simulink model "threephase_matrix_converter"  (R2014a)
settings: Solver=ode23tb  StartTime=0.0  StopTime=0.1  RelTol=1e-4
PreLoadFcn:
  | Ts=2.5e-6;
InitFcn:
  | Ts=2.5e-6;
StartFcn:
  | tic;
StopFcn:
  | toc;
undefined symbols (not defined in the file or in its folder): DiscIntNeverNeededParam
libraries: powerlib x46, simulink x6
(part 1 of 2)
Description:
  | Copyright 2008 The MathWorks(TM), Inc.
settings Model: Creator=Graham Dudgeon  LastModifiedBy=cosorio
settings DataIOCC: SaveOutput=off  SaveTime=off
settings OptimizationCC: ExpressionDepthLimit=2147483647  InitFltsAndDblsToZero=on
settings DebuggingCC: SaveWithParameterizedLinksMsg=none  UnderspecifiedInitializationDetection=Classic  SignalResolutionControl=TryResolveAllWithWarning  SolverPrmCheckMsg=none  MultiTaskDSMMsg=warning  MultiTaskCondExecSysMsg=none  FcnCallInpInsideContextMsg=UseLocalSettings  StateNameClashWarn=warning
settings RTWCC: IncludeERTFirstTime=on
settings GRTTargetCC: TargetFcnLib=ansi_tfl_tmw.mat  CombineOutputUpdateFcns=off  GRTInterface=on

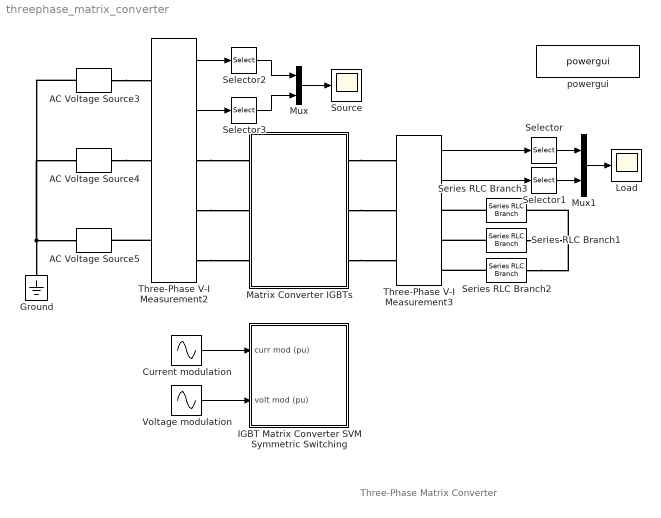
== system threephase_matrix_converter ==
  note: Three-Phase Matrix Converter
  AC Voltage Source3 : powerlib/Electrical Sources/AC Voltage Source  Amplitude=100  Phase=0  Frequency=60  SampleTime=0  Measurements=None
  AC Voltage Source4 : powerlib/Electrical Sources/AC Voltage Source  Amplitude=100  Phase=-120  Frequency=60  SampleTime=0  Measurements=None
  AC Voltage Source5 : powerlib/Electrical Sources/AC Voltage Source  Amplitude=100  Phase=120  Frequency=60  SampleTime=0  Measurements=None
  Current modulation : Sin  Amplitude=1*sqrt(2)/sqrt(3)  Frequency=2*pi*60  Phase=[0 -2*pi/3 2*pi/3]  SampleTime=0
  Ground : powerlib/Elements/Ground  LConnTagsString=a
  IGBT Matrix Converter SVM Symmetric Switching : Subsystem
  Load : Scope
      settings: YMin=-175  YMax=175  SaveName=vl1
  Matrix Converter IGBTs : Subsystem
      mask Display:
      | plot([0 10],[0 0])
      | plot([0 10],[4 4])
      | plot([0 10],[8 8])
      | plot([10 11],[8 7],[11 12.5],[7 6.5],[12 13],[6 5])
      | plot([10 11]-4,[8 7],[11 12.5]-4,[7 6.5],[12 13]-4,[6 5])
      | plot([10 11]-8,[8 7],[11 12.5]-8,[7 6.5],[12 13]-8,[6 5])
      | plot([10 11],[8 7]-4,[11 12.5],[7 6.5]-4,[12 13],[6 5]-4)
      | plot([10 11]-4,[8 7]-4,[11 12.5]-4,[7 6.5]-4,[12 13]-4,[6 5]-4)
      | plot([10 11]-8,[8 7]-4,[11 12.5]-8,[7 6.5]-4,[12 13]-8,[6 5]-4)
      | plot([10 11],[8 7]-8,[11 12.5],[7 6.5]-8,[12 13],[6 5]-8)
      | plot([10 11]-4,[8 7]-8,[11 12.5]-4,[7 6.5]-8,[12 13]-4,[6 5]-8)
      | plot([10 11]-8,[8 7]-8,[11 12.5]-8,[7 6.5]-8,[12 13]-8,[6 5]-8)
      | plot([5 5],[-5 5])
      | plot([9 9],[-5 5])
      | plot([13 13],[-5 5])
      | plot(-2,-6,15,9)
      | plot([0 0],[-5 -2])
      | plot([0.5 0.5],[-5 -2])
      | plot([0.5 1.5],[-4 -5])
      | plot([0.5 1.5],[-3 -2])
      | plot([1.5 1.5],[-5 -6])
      | plot([1.5 1.5],[-2 -1])
      | plot([1 1.5],[-4.8 -5])
      | plot([1.3 1.5],[-4.4 -5])
      | plot([-0.5 0],[-5 -5])
  Mux : Mux  Inputs=2
  Mux1 : Mux  Inputs=2
  Selector{,1..3} (4 alike) : Selector  InputPortWidth=3
  Series RLC Branch1 : powerlib/Elements/Series RLC Branch  LConnTagsString=__new0  RConnTagsString=__new0  BranchType=R  Resistance=2  Inductance=1e-3  SetiL0=off  InitialCurrent=0  Capacitance=[]  Setx0=off  InitialVoltage=0  Measurements=None
  Series RLC Branch2 : powerlib/Elements/Series RLC Branch  LConnTagsString=__new0  RConnTagsString=__new0  BranchType=R  Resistance=2  Inductance=1e-3  SetiL0=off  InitialCurrent=0  Capacitance=[]  Setx0=off  InitialVoltage=0  Measurements=None
  Series RLC Branch3 : powerlib/Elements/Series RLC Branch  LConnTagsString=__new0  RConnTagsString=__new0  BranchType=R  Resistance=2  Inductance=1e-3  SetiL0=off  InitialCurrent=0  Capacitance=[]  Setx0=off  InitialVoltage=0  Measurements=None
  Source : Scope
      settings: YMin=-100  YMax=100  SaveName=vl
  Three-Phase V-I Measurement2 : powerlib/Measurements/Three-Phase V-I Measurement  VoltageMeasurement=phase-to-ground  SetLabelV=off  LabelV=Vabc  Vpu=off  VpuLL=off  CurrentMeasurement=yes  SetLabelI=off  LabelI=Iabc  Ipu=off  Pbase=100e6  Vbase=500e3  OutputType=Complex  PhasorSimulation=off  PSBequivalent=0
  Three-Phase V-I Measurement3 : powerlib/Measurements/Three-Phase V-I Measurement  VoltageMeasurement=phase-to-phase  SetLabelV=off  LabelV=Vabc  Vpu=off  VpuLL=off  CurrentMeasurement=yes  SetLabelI=off  LabelI=Iabc  Ipu=off  Pbase=100e6  Vbase=500e3  OutputType=Complex  PhasorSimulation=off  PSBequivalent=0
  Voltage modulation : Sin  Amplitude=1*sqrt(2)/sqrt(3)  Frequency=2*pi*60  Phase=[0 -2*pi/3 2*pi/3]  SampleTime=0
  powergui : powerlib/powergui  SimulationMode=Continuous  SolverType=Tustin  SampleTime=2.5e-6  frequency=60  SPID=off  DisableSnubberDevices=on  DisableRonSwitches=off  DisableVfSwitches=off  SwTol=0  Interpol=off  DisplayEquations=off  Ts=0  methode=off  frequencyindice=60  Pbase=100e6  ErrMax=1e-4  Iterations=50  UnitsV=kV  UnitsW=MW  FunctionMessages=off  echomessages=off  HookPort=off  EnableUseOfTLC=off  x0status=blocks  RestoreLinks=warning  ResistiveCurrentMeasurement=off  Frange=[0:2:500]  Ylog=off  Xlog=on  ShowGrid=off  save=off  variable=ZData  structure=Vs  ZoomFFT=on  StartTime=1/60  cycles=1  DisplayStyle=1  fundamental=60  FreqAxis=on  MaxFrequency=10000  frequencyindicesteady=1  RmsSteady=1  display=off
  wires:
  Current modulation/1 -> IGBT Matrix Converter SVM Symmetric Switching/1(curr mod (pu))
  Voltage modulation/1 -> IGBT Matrix Converter SVM Symmetric Switching/2(volt mod (pu))
  Three-Phase V-I Measurement3/1 -> Selector/1
  Three-Phase V-I Measurement3/2 -> Selector1/1
  Selector/1 -> Mux1/1
  Three-Phase V-I Measurement2/1 -> Selector2/1
  Three-Phase V-I Measurement2/2 -> Selector3/1
  Selector2/1 -> Mux/1
  Selector3/1 -> Mux/2
  Mux/1 -> Source/1
  Selector1/1 -> Mux1/2
  Mux1/1 -> Load/1
  connections:
  AC Voltage Source4/LConn1 -- AC Voltage Source3/LConn1 -- Ground/LConn1 -- AC Voltage Source5/LConn1
  Three-Phase V-I Measurement2/RConn1 -- Matrix Converter IGBTs/LConn1
  Three-Phase V-I Measurement2/RConn3 -- Matrix Converter IGBTs/LConn3
  AC Voltage Source3/RConn1 -- Three-Phase V-I Measurement2/LConn1
  Three-Phase V-I Measurement2/LConn3 -- AC Voltage Source5/RConn1
  AC Voltage Source4/RConn1 -- Three-Phase V-I Measurement2/LConn2
  Three-Phase V-I Measurement2/RConn2 -- Matrix Converter IGBTs/LConn2
  Series RLC Branch2/RConn1 -- Series RLC Branch1/RConn1 -- Series RLC Branch3/RConn1
  Series RLC Branch3/LConn1 -- Three-Phase V-I Measurement3/RConn1
  Series RLC Branch1/LConn1 -- Three-Phase V-I Measurement3/RConn2
  Series RLC Branch2/LConn1 -- Three-Phase V-I Measurement3/RConn3
  Matrix Converter IGBTs/RConn2 -- Three-Phase V-I Measurement3/LConn2
  Matrix Converter IGBTs/RConn3 -- Three-Phase V-I Measurement3/LConn3
  Matrix Converter IGBTs/RConn1 -- Three-Phase V-I Measurement3/LConn1

== system threephase_matrix_converter/IGBT Matrix Converter SVM Symmetric Switching ==
  curr mod (pu) : Inport
  volt mod (pu) : Inport  Port=2
  SVM Inversion symmetric sequence : Subsystem  mask{switching_freq=6000}
      mask prompts: switching_freq "switching frequency (Hz)"
  SVM Rectification symmetric sequence : Subsystem  mask{switching_freq=6000}
      mask prompts: switching_freq "switching frequency (Hz)"
  Scope{1..6} (6 alike) : Scope
      Scope1 settings: TimeRange=0.1  YMin=1000  YMax=8000  SaveName=Vabc  Decimation=100
      Scope2 settings: TimeRange=0.1  YMin=1000  YMax=8000  SaveName=Vabc1  Decimation=100
      Scope3 settings: TimeRange=0.1  YMin=1000  YMax=8000  SaveName=Vabc2  Decimation=100
      Scope4 settings: TimeRange=0.1  YMin=1000  YMax=8000  SaveName=Vabc3  Decimation=100
      Scope5 settings: TimeRange=0.1  YMin=1000  YMax=8000  SaveName=Vabc4  Decimation=100
      Scope6 settings: TimeRange=0.1  YMin=1000  YMax=8000  SaveName=Vabc5  Decimation=100
  matrix converter switching : Subsystem
  matrix-converter switching count : Subsystem
  six-device switching count : Subsystem
  six-device switching count1 : Subsystem
  wires:
  SVM Inversion symmetric sequence/1(g) -> matrix converter switching/2(gI), six-device switching count1/1(pulses)
  SVM Rectification symmetric sequence/1(g) -> matrix converter switching/1(gR), six-device switching count/1(pulses)
  curr mod (pu)/1 -> SVM Rectification symmetric sequence/1(mod (pu))
  volt mod (pu)/1 -> SVM Inversion symmetric sequence/1(mod (pu))
  matrix-converter switching count/2(individual) -> Scope2/1
  matrix-converter switching count/1(total) -> Scope1/1
  matrix converter switching/1(g) -> matrix-converter switching count/1(pulses)
  six-device switching count/1(total) -> Scope3/1
  six-device switching count/2(individual) -> Scope4/1
  six-device switching count1/1(total) -> Scope5/1
  six-device switching count1/2(individual) -> Scope6/1

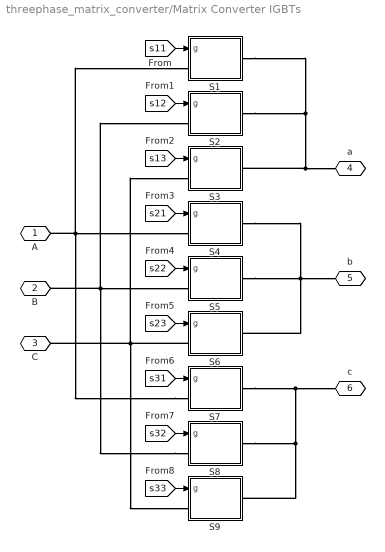
== system threephase_matrix_converter/Matrix Converter IGBTs ==
  S1 : Subsystem
  S2 : Subsystem
  S3 : Subsystem
  S4 : Subsystem
  S5 : Subsystem
  S6 : Subsystem
  S7 : Subsystem
  S8 : Subsystem
  S9 : Subsystem
  A : PMIOPort  Port=1  Side=Left
  B : PMIOPort  Port=2  Side=Left
  C : PMIOPort  Port=3  Side=Left
  a : PMIOPort  Port=4  Side=Right
  b : PMIOPort  Port=5  Side=Right
  c : PMIOPort  Port=6  Side=Right
  wires:
  [s33] -> S9/1(g)
  [s32] -> S8/1(g)
  [s31] -> S7/1(g)
  [s23] -> S6/1(g)
  [s22] -> S5/1(g)
  [s21] -> S4/1(g)
  [s13] -> S3/1(g)
  [s12] -> S2/1(g)
  [s11] -> S1/1(g)
  connections:
  c/RConn1 -- S7/RConn1 -- S9/RConn1 -- S8/RConn1
  S6/RConn1 -- S4/RConn1 -- b/RConn1 -- S5/RConn1
  C/RConn1 -- S3/LConn1 -- S6/LConn1 -- S9/LConn1
  S8/LConn1 -- S2/LConn1 -- B/RConn1 -- S5/LConn1
  S3/RConn1 -- S1/RConn1 -- S2/RConn1 -- a/RConn1
  S7/LConn1 -- A/RConn1 -- S1/LConn1 -- S4/LConn1

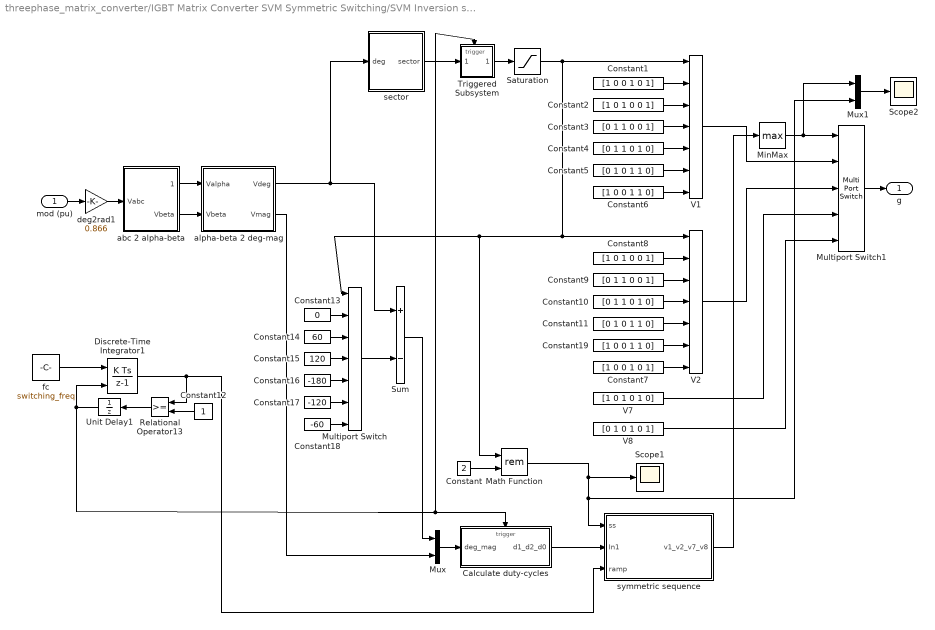
== system threephase_matrix_converter/IGBT Matrix Converter SVM Symmetric Switching/SVM Inversion symmetric sequence ==
  mod (pu) : Inport
  Calculate duty-cycles : Subsystem  TreatAsAtomicUnit=on
  Constant : Constant  Value=2
  Constant1 : Constant  Value=[1 0 0 1 0 1]
  Constant10 : Constant  Value=[0 1 1 0 1 0]
  Constant11 : Constant  Value=[0 1 0 1 1 0]
  Constant12 : Constant
  Constant13 : Constant  Value=0
  Constant14 : Constant  Value=60
  Constant15 : Constant  Value=120
  Constant16 : Constant  Value=-180
  Constant17 : Constant  Value=-120
  Constant18 : Constant  Value=-60
  Constant19 : Constant  Value=[1 0 0 1 1 0]
  Constant2 : Constant  Value=[1 0 1 0 0 1]
  Constant3 : Constant  Value=[0 1 1 0 0 1]
  Constant4 : Constant  Value=[0 1 1 0 1 0]
  Constant5 : Constant  Value=[0 1 0 1 1 0]
  Constant6 : Constant  Value=[1 0 0 1 1 0]
  Constant7 : Constant  Value=[1 0 0 1 0 1]
  Constant8 : Constant  Value=[1 0 1 0 0 1]
  Constant9 : Constant  Value=[0 1 1 0 0 1]
  Discrete-Time Integrator1 : DiscreteIntegrator  ExternalReset=rising  SampleTime=Ts  ICPrevOutput=DiscIntNeverNeededParam  ICPrevScaledInput=DiscIntNeverNeededParam
  Math Function : Math  Operator=rem  SaturateOnIntegerOverflow=on
  MinMax : MinMax  Function=max
  Multiport Switch : MultiPortSwitch  Inputs=6
  Multiport Switch1 : MultiPortSwitch  Inputs=4
  Mux : Mux  Inputs=2
  Mux1 : Mux  Inputs=2
  Relational Operator13 : RelationalOperator  InputSameDT=on
  Saturation : Saturate  UpperLimit=6  LowerLimit=1
  Scope1 : Scope
      settings: YMin=-0.1  YMax=4.1  SaveName=Iabc1
  Scope2 : Scope
      settings: YMin=-0.1  YMax=4.1  SaveName=Iabc2
  Sum : Sum  Inputs=+-
  Triggered Subsystem : Subsystem  TreatAsAtomicUnit=on
  Unit Delay1 : UnitDelay  SampleTime=Ts
  V1 : MultiPortSwitch  Inputs=6
  V2 : MultiPortSwitch  Inputs=6
  V7 : Constant  Value=[1 0 1 0 1 0]
  V8 : Constant  Value=[0 1 0 1 0 1]
  abc 2 alpha-beta : Subsystem
  alpha-beta 2 deg-mag : Subsystem
  deg2rad1 : Gain  Gain=0.866
  fc : Constant  Value=switching_freq
  sector : Subsystem
  symmetric sequence : Subsystem
  g : Outport
  wires:
  Mux1/1 -> Scope2/1
  Math Function/1 -> Mux1/2, symmetric sequence/1(ss), Scope1/1
  symmetric sequence/1(v1_v2_v7_v8) -> MinMax/1
  Constant/1 -> Math Function/2
  deg2rad1/1 -> abc 2 alpha-beta/1(Vabc)
  Triggered Subsystem/1(Out1) -> Saturation/1
  sector/1(sector) -> Triggered Subsystem/1(In1)
  Saturation/1 -> V1/1, Math Function/1, Multiport Switch/1, V2/1
  Unit Delay1/1 -> Calculate duty-cycles/Trigger, Triggered Subsystem/Trigger, Discrete-Time Integrator1/2
  Multiport Switch1/1 -> g/1
  MinMax/1 -> Mux1/1, Multiport Switch1/1
  V8/1 -> Multiport Switch1/5
  V7/1 -> Multiport Switch1/4
  V2/1 -> Multiport Switch1/3
  V1/1 -> Multiport Switch1/2
  Constant7/1 -> V2/7
  Constant6/1 -> V1/7
  Constant2/1 -> V1/3
  Constant19/1 -> V2/6
  Constant11/1 -> V2/5
  Constant10/1 -> V2/4
  Constant9/1 -> V2/3
  Constant8/1 -> V2/2
  Constant5/1 -> V1/6
  Constant4/1 -> V1/5
  Constant3/1 -> V1/4
  Constant1/1 -> V1/2
  Sum/1 -> Mux/1
  Multiport Switch/1 -> Sum/2
  Constant18/1 -> Multiport Switch/7
  Constant17/1 -> Multiport Switch/6
  Constant16/1 -> Multiport Switch/5
  Constant15/1 -> Multiport Switch/4
  Constant14/1 -> Multiport Switch/3
  Constant13/1 -> Multiport Switch/2
  Calculate duty-cycles/1(d1_d2_d0) -> symmetric sequence/2(In1)
  abc 2 alpha-beta/2(Vbeta) -> alpha-beta 2 deg-mag/2(Vbeta)
  abc 2 alpha-beta/1(Valpha) -> alpha-beta 2 deg-mag/1(Valpha)
  Mux/1 -> Calculate duty-cycles/1(deg_mag)
  fc/1 -> Discrete-Time Integrator1/1
  Discrete-Time Integrator1/1 -> symmetric sequence/3(ramp), Relational Operator13/1
  Constant12/1 -> Relational Operator13/2
  Relational Operator13/1 -> Unit Delay1/1
  alpha-beta 2 deg-mag/2(Vmag) -> Mux/2
  alpha-beta 2 deg-mag/1(Vdeg) -> sector/1(deg), Sum/1
  mod (pu)/1 -> deg2rad1/1

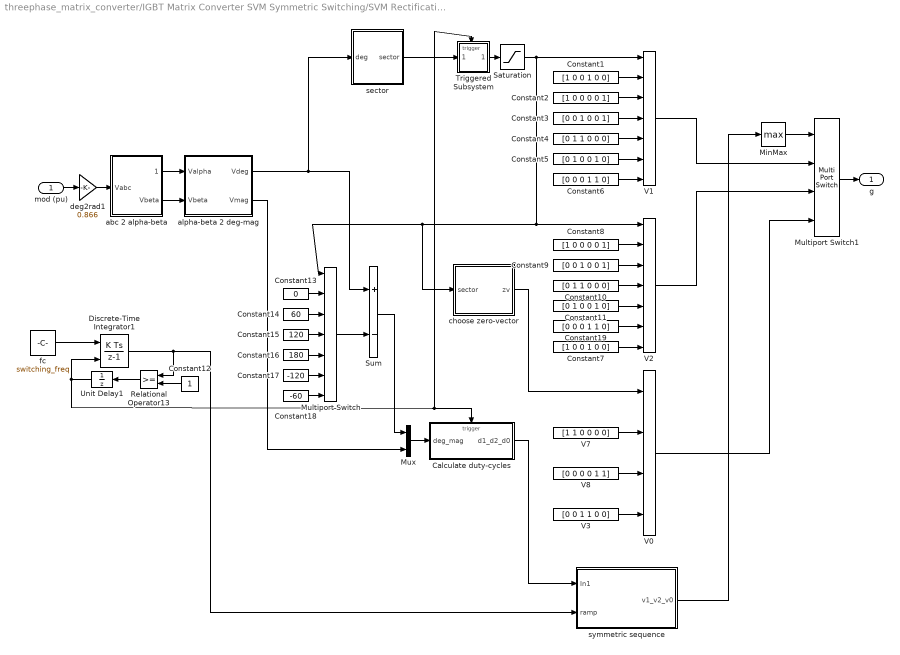
== system threephase_matrix_converter/IGBT Matrix Converter SVM Symmetric Switching/SVM Rectification symmetric sequence ==
  mod (pu) : Inport
  Calculate duty-cycles : Subsystem  TreatAsAtomicUnit=on
  Constant1 : Constant  Value=[1 0 0 1 0 0]
  Constant10 : Constant  Value=[0 1 1 0 0 0]
  Constant11 : Constant  Value=[0 1 0 0 1 0]
  Constant12 : Constant
  Constant13 : Constant  Value=0
  Constant14 : Constant  Value=60
  Constant15 : Constant  Value=120
  Constant16 : Constant  Value=180
  Constant17 : Constant  Value=-120
  Constant18 : Constant  Value=-60
  Constant19 : Constant  Value=[0 0 0 1 1 0]
  Constant2 : Constant  Value=[1 0 0 0 0 1]
  Constant3 : Constant  Value=[0 0 1 0 0 1]
  Constant4 : Constant  Value=[0 1 1 0 0 0]
  Constant5 : Constant  Value=[0 1 0 0 1 0]
  Constant6 : Constant  Value=[0 0 0 1 1 0]
  Constant7 : Constant  Value=[1 0 0 1 0 0]
  Constant8 : Constant  Value=[1 0 0 0 0 1]
  Constant9 : Constant  Value=[0 0 1 0 0 1]
  Discrete-Time Integrator1 : DiscreteIntegrator  ExternalReset=rising  SampleTime=Ts  ICPrevOutput=DiscIntNeverNeededParam  ICPrevScaledInput=DiscIntNeverNeededParam
  MinMax : MinMax  Function=max
  Multiport Switch : MultiPortSwitch  Inputs=6
  Multiport Switch1 : MultiPortSwitch
  Mux : Mux  Inputs=2
  Relational Operator13 : RelationalOperator  InputSameDT=on
  Saturation : Saturate  UpperLimit=6  LowerLimit=1
  Sum : Sum  Inputs=+-
  Triggered Subsystem : Subsystem  TreatAsAtomicUnit=on
  Unit Delay1 : UnitDelay  SampleTime=Ts
  V0 : MultiPortSwitch
  V1 : MultiPortSwitch  Inputs=6
  V2 : MultiPortSwitch  Inputs=6
  V3 : Constant  Value=[0 0 1 1 0 0]
  V7 : Constant  Value=[1 1 0 0 0 0]
  V8 : Constant  Value=[0 0 0 0 1 1]
  abc 2 alpha-beta : Subsystem
  alpha-beta 2 deg-mag : Subsystem
  choose zero-vector : Subsystem
  deg2rad1 : Gain  Gain=0.866
  fc : Constant  Value=switching_freq
  sector : Subsystem
  symmetric sequence : Subsystem
  g : Outport
  wires:
  deg2rad1/1 -> abc 2 alpha-beta/1(Vabc)
  Saturation/1 -> V1/1, V2/1, Multiport Switch/1, choose zero-vector/1(sector)
  Triggered Subsystem/1(Out1) -> Saturation/1
  sector/1(sector) -> Triggered Subsystem/1(In1)
  MinMax/1 -> Multiport Switch1/1
  Unit Delay1/1 -> Discrete-Time Integrator1/2, Calculate duty-cycles/Trigger, Triggered Subsystem/Trigger
  Multiport Switch1/1 -> g/1
  symmetric sequence/1(v1_v2_v0) -> MinMax/1
  V2/1 -> Multiport Switch1/3
  V1/1 -> Multiport Switch1/2
  Constant7/1 -> V2/7
  Constant6/1 -> V1/7
  Constant2/1 -> V1/3
  Constant19/1 -> V2/6
  Constant11/1 -> V2/5
  Constant10/1 -> V2/4
  Constant9/1 -> V2/3
  Constant8/1 -> V2/2
  Constant5/1 -> V1/6
  Constant4/1 -> V1/5
  Constant3/1 -> V1/4
  Constant1/1 -> V1/2
  Sum/1 -> Mux/1
  Multiport Switch/1 -> Sum/2
  Constant18/1 -> Multiport Switch/7
  Constant17/1 -> Multiport Switch/6
  Constant16/1 -> Multiport Switch/5
  Constant15/1 -> Multiport Switch/4
  Constant14/1 -> Multiport Switch/3
  Constant13/1 -> Multiport Switch/2
  Calculate duty-cycles/1(d1_d2_d0) -> symmetric sequence/1(In1)
  abc 2 alpha-beta/2(Vbeta) -> alpha-beta 2 deg-mag/2(Vbeta)
  abc 2 alpha-beta/1(Valpha) -> alpha-beta 2 deg-mag/1(Valpha)
  Mux/1 -> Calculate duty-cycles/1(deg_mag)
  fc/1 -> Discrete-Time Integrator1/1
  Discrete-Time Integrator1/1 -> Relational Operator13/1, symmetric sequence/2(ramp)
  Constant12/1 -> Relational Operator13/2
  Relational Operator13/1 -> Unit Delay1/1
  alpha-beta 2 deg-mag/2(Vmag) -> Mux/2
  alpha-beta 2 deg-mag/1(Vdeg) -> sector/1(deg), Sum/1
  mod (pu)/1 -> deg2rad1/1
  V7/1 -> V0/2
  V8/1 -> V0/3
  V3/1 -> V0/4
  V0/1 -> Multiport Switch1/4
  choose zero-vector/1(zv) -> V0/1

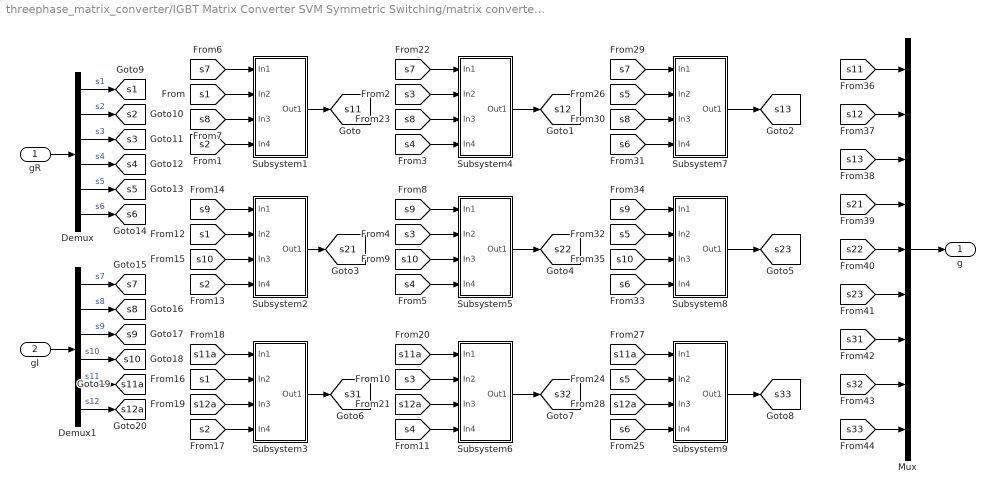
== system threephase_matrix_converter/IGBT Matrix Converter SVM Symmetric Switching/matrix converter switching ==
  gR : Inport
  gI : Inport  Port=2
  Demux : Demux  Outputs=6
  Demux1 : Demux  Outputs=6
  Mux : Mux  Inputs=9
  Subsystem1 : Subsystem
  Subsystem2 : Subsystem
  Subsystem3 : Subsystem
  Subsystem4 : Subsystem
  Subsystem5 : Subsystem
  Subsystem6 : Subsystem
  Subsystem7 : Subsystem
  Subsystem8 : Subsystem
  Subsystem9 : Subsystem
  g : Outport
  tag scope: s10=global, s11=global, s11a=global, s12=global, s12a=global, s13=global, s1=global, s21=global, s22=global, s23=global, s2=global, s31=global, s32=global, s33=global, s3=global, s4=global, s5=global, s6=global, s7=global, s8=global, s9=global
  wires:
  Demux/4 -> [s4]  "s4"
  Demux1/6 -> [s12a]  "s12"
  gR/1 -> Demux/1
  gI/1 -> Demux1/1
  Demux/1 -> [s1]  "s1"
  Demux1/5 -> [s11a]  "s11"
  Demux1/4 -> [s10]  "s10"
  Demux1/3 -> [s9]  "s9"
  Demux1/2 -> [s8]  "s8"
  Demux1/1 -> [s7]  "s7"
  Demux/2 -> [s2]  "s2"
  Demux/3 -> [s3]  "s3"
  Demux/5 -> [s5]  "s5"
  Demux/6 -> [s6]  "s6"
  [s7] -> Subsystem1/1(In1)
  [s1] -> Subsystem1/2(In2)
  [s8] -> Subsystem1/3(In3)
  [s2] -> Subsystem1/4(In4)
  [s9] -> Subsystem2/1(In1)
  [s1] -> Subsystem2/2(In2)
  [s10] -> Subsystem2/3(In3)
  [s2] -> Subsystem2/4(In4)
  [s11a] -> Subsystem3/1(In1)
  [s1] -> Subsystem3/2(In2)
  [s12a] -> Subsystem3/3(In3)
  [s2] -> Subsystem3/4(In4)
  [s7] -> Subsystem4/1(In1)
  [s3] -> Subsystem4/2(In2)
  [s8] -> Subsystem4/3(In3)
  [s4] -> Subsystem4/4(In4)
  [s9] -> Subsystem5/1(In1)
  [s3] -> Subsystem5/2(In2)
  [s10] -> Subsystem5/3(In3)
  [s4] -> Subsystem5/4(In4)
  [s11a] -> Subsystem6/1(In1)
  [s3] -> Subsystem6/2(In2)
  [s12a] -> Subsystem6/3(In3)
  [s4] -> Subsystem6/4(In4)
  [s7] -> Subsystem7/1(In1)
  [s5] -> Subsystem7/2(In2)
  [s8] -> Subsystem7/3(In3)
  [s6] -> Subsystem7/4(In4)
  [s9] -> Subsystem8/1(In1)
  [s5] -> Subsystem8/2(In2)
  [s10] -> Subsystem8/3(In3)
  [s6] -> Subsystem8/4(In4)
  [s11a] -> Subsystem9/1(In1)
  [s5] -> Subsystem9/2(In2)
  [s12a] -> Subsystem9/3(In3)
  [s6] -> Subsystem9/4(In4)
  Subsystem1/1(Out1) -> [s11]
  Subsystem4/1(Out1) -> [s12]
  Subsystem7/1(Out1) -> [s13]
  Subsystem2/1(Out1) -> [s21]
  Subsystem5/1(Out1) -> [s22]
  Subsystem8/1(Out1) -> [s23]
  Subsystem3/1(Out1) -> [s31]
  Subsystem6/1(Out1) -> [s32]
  Subsystem9/1(Out1) -> [s33]
  [s11] -> Mux/1
  [s12] -> Mux/2
  [s13] -> Mux/3
  [s21] -> Mux/4
  [s22] -> Mux/5
  [s23] -> Mux/6
  [s31] -> Mux/7
  [s32] -> Mux/8
  [s33] -> Mux/9
  Mux/1 -> g/1

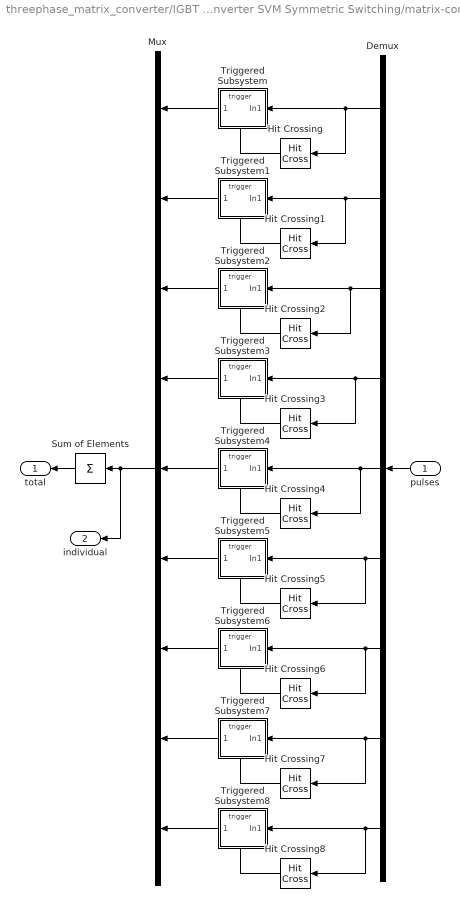
== system threephase_matrix_converter/IGBT Matrix Converter SVM Symmetric Switching/matrix-converter switching count ==
  pulses : Inport
  Demux : Demux  Outputs=9
  Hit Crossing{,1..8} (9 alike) : HitCross  HitCrossingDirection=rising
  Mux : Mux  Inputs=9
  Sum of Elements : Sum  Inputs=+
  Triggered Subsystem : Subsystem  TreatAsAtomicUnit=on
  Triggered Subsystem1 : Subsystem  TreatAsAtomicUnit=on
  Triggered Subsystem2 : Subsystem  TreatAsAtomicUnit=on
  Triggered Subsystem3 : Subsystem  TreatAsAtomicUnit=on
  Triggered Subsystem4 : Subsystem  TreatAsAtomicUnit=on
  Triggered Subsystem5 : Subsystem  TreatAsAtomicUnit=on
  Triggered Subsystem6 : Subsystem  TreatAsAtomicUnit=on
  Triggered Subsystem7 : Subsystem  TreatAsAtomicUnit=on
  Triggered Subsystem8 : Subsystem  TreatAsAtomicUnit=on
  total : Outport
  individual : Outport  Port=2
  wires:
  pulses/1 -> Demux/1
  Sum of Elements/1 -> total/1
  Mux/1 -> individual/1, Sum of Elements/1
  Demux/6 -> Triggered Subsystem5/1(In1), Hit Crossing5/1
  Hit Crossing5/1 -> Triggered Subsystem5/Trigger
  Triggered Subsystem5/1(Out1) -> Mux/6
  Demux/5 -> Triggered Subsystem4/1(In1), Hit Crossing4/1
  Hit Crossing4/1 -> Triggered Subsystem4/Trigger
  Triggered Subsystem4/1(Out1) -> Mux/5
  Demux/4 -> Triggered Subsystem3/1(In1), Hit Crossing3/1
  Hit Crossing3/1 -> Triggered Subsystem3/Trigger
  Triggered Subsystem3/1(Out1) -> Mux/4
  Demux/3 -> Triggered Subsystem2/1(In1), Hit Crossing2/1
  Hit Crossing2/1 -> Triggered Subsystem2/Trigger
  Triggered Subsystem2/1(Out1) -> Mux/3
  Demux/2 -> Triggered Subsystem1/1(In1), Hit Crossing1/1
  Hit Crossing1/1 -> Triggered Subsystem1/Trigger
  Triggered Subsystem1/1(Out1) -> Mux/2
  Demux/1 -> Triggered Subsystem/1(In1), Hit Crossing/1
  Hit Crossing/1 -> Triggered Subsystem/Trigger
  Triggered Subsystem/1(Out1) -> Mux/1
  Demux/7 -> Triggered Subsystem6/1(In1), Hit Crossing6/1
  Hit Crossing6/1 -> Triggered Subsystem6/Trigger
  Triggered Subsystem6/1(Out1) -> Mux/7
  Demux/8 -> Triggered Subsystem7/1(In1), Hit Crossing7/1
  Hit Crossing7/1 -> Triggered Subsystem7/Trigger
  Triggered Subsystem7/1(Out1) -> Mux/8
  Demux/9 -> Triggered Subsystem8/1(In1), Hit Crossing8/1
  Hit Crossing8/1 -> Triggered Subsystem8/Trigger
  Triggered Subsystem8/1(Out1) -> Mux/9

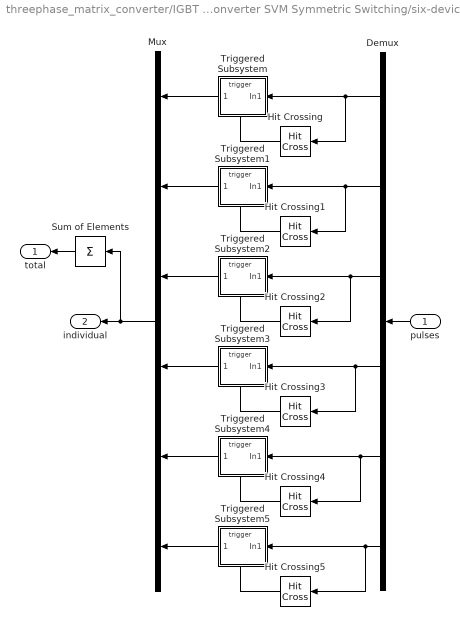
== system threephase_matrix_converter/IGBT Matrix Converter SVM Symmetric Switching/six-device switching count ==
  pulses : Inport
  Demux : Demux  Outputs=6
  Hit Crossing{,1..5} (6 alike) : HitCross  HitCrossingDirection=rising
  Mux : Mux  Inputs=6
  Sum of Elements : Sum  Inputs=+
  Triggered Subsystem : Subsystem  TreatAsAtomicUnit=on
  Triggered Subsystem1 : Subsystem  TreatAsAtomicUnit=on
  Triggered Subsystem2 : Subsystem  TreatAsAtomicUnit=on
  Triggered Subsystem3 : Subsystem  TreatAsAtomicUnit=on
  Triggered Subsystem4 : Subsystem  TreatAsAtomicUnit=on
  Triggered Subsystem5 : Subsystem  TreatAsAtomicUnit=on
  total : Outport
  individual : Outport  Port=2
  wires:
  pulses/1 -> Demux/1
  Sum of Elements/1 -> total/1
  Mux/1 -> individual/1, Sum of Elements/1
  Demux/6 -> Triggered Subsystem5/1(In1), Hit Crossing5/1
  Hit Crossing5/1 -> Triggered Subsystem5/Trigger
  Triggered Subsystem5/1(Out1) -> Mux/6
  Demux/5 -> Triggered Subsystem4/1(In1), Hit Crossing4/1
  Hit Crossing4/1 -> Triggered Subsystem4/Trigger
  Triggered Subsystem4/1(Out1) -> Mux/5
  Demux/4 -> Triggered Subsystem3/1(In1), Hit Crossing3/1
  Hit Crossing3/1 -> Triggered Subsystem3/Trigger
  Triggered Subsystem3/1(Out1) -> Mux/4
  Demux/3 -> Triggered Subsystem2/1(In1), Hit Crossing2/1
  Hit Crossing2/1 -> Triggered Subsystem2/Trigger
  Triggered Subsystem2/1(Out1) -> Mux/3
  Demux/2 -> Triggered Subsystem1/1(In1), Hit Crossing1/1
  Hit Crossing1/1 -> Triggered Subsystem1/Trigger
  Triggered Subsystem1/1(Out1) -> Mux/2
  Demux/1 -> Triggered Subsystem/1(In1), Hit Crossing/1
  Hit Crossing/1 -> Triggered Subsystem/Trigger
  Triggered Subsystem/1(Out1) -> Mux/1

== system threephase_matrix_converter/IGBT Matrix Converter SVM Symmetric Switching/six-device switching count1 ==
  pulses : Inport
  Demux : Demux  Outputs=6
  Hit Crossing{,1..5} (6 alike) : HitCross  HitCrossingDirection=rising
  Mux : Mux  Inputs=6
  Sum of Elements : Sum  Inputs=+
  Triggered Subsystem : Subsystem  TreatAsAtomicUnit=on
  Triggered Subsystem1 : Subsystem  TreatAsAtomicUnit=on
  Triggered Subsystem2 : Subsystem  TreatAsAtomicUnit=on
  Triggered Subsystem3 : Subsystem  TreatAsAtomicUnit=on
  Triggered Subsystem4 : Subsystem  TreatAsAtomicUnit=on
  Triggered Subsystem5 : Subsystem  TreatAsAtomicUnit=on
  total : Outport
  individual : Outport  Port=2
  wires:
  Triggered Subsystem/1(Out1) -> Mux/1
  Hit Crossing/1 -> Triggered Subsystem/Trigger
  Demux/1 -> Hit Crossing/1, Triggered Subsystem/1(In1)
  Triggered Subsystem1/1(Out1) -> Mux/2
  Hit Crossing1/1 -> Triggered Subsystem1/Trigger
  Demux/2 -> Hit Crossing1/1, Triggered Subsystem1/1(In1)
  Triggered Subsystem2/1(Out1) -> Mux/3
  Hit Crossing2/1 -> Triggered Subsystem2/Trigger
  Demux/3 -> Hit Crossing2/1, Triggered Subsystem2/1(In1)
  Triggered Subsystem3/1(Out1) -> Mux/4
  Hit Crossing3/1 -> Triggered Subsystem3/Trigger
  Demux/4 -> Hit Crossing3/1, Triggered Subsystem3/1(In1)
  Triggered Subsystem4/1(Out1) -> Mux/5
  Hit Crossing4/1 -> Triggered Subsystem4/Trigger
  Demux/5 -> Hit Crossing4/1, Triggered Subsystem4/1(In1)
  Triggered Subsystem5/1(Out1) -> Mux/6
  Hit Crossing5/1 -> Triggered Subsystem5/Trigger
  Demux/6 -> Hit Crossing5/1, Triggered Subsystem5/1(In1)
  Mux/1 -> Sum of Elements/1, individual/1
  Sum of Elements/1 -> total/1
  pulses/1 -> Demux/1

== system threephase_matrix_converter/Matrix Converter IGBTs/S1 ==
  g : Inport
  Diode : powerlib/Power Electronics/Diode  Ron=0.001  Lon=0  Vf=0  IC=0  UseSnubber=off  Rs=1e4  Cs=250e-9  Measurements=off
  Diode1 : powerlib/Power Electronics/Diode  Ron=0.001  Lon=0  Vf=0  IC=0  UseSnubber=off  Rs=1e4  Cs=250e-9  Measurements=off
  IGBT1 : powerlib/Power Electronics/IGBT  Ron=0.001  Lon=0  Vf=1  Tf=1e-6  Tt=2e-6  IC=0  Rs=1e5  Cs=inf  Measurements=off
  IGBT2 : powerlib/Power Electronics/IGBT  Ron=0.001  Lon=0  Vf=1  Tf=1e-6  Tt=2e-6  IC=0  Rs=1e5  Cs=inf  Measurements=off
  + : PMIOPort  Port=1  Side=Left
  - : PMIOPort  Port=2  Side=Right
  wires:
  g/1 -> IGBT2/1, IGBT1/1
  connections:
  IGBT2/LConn1 -- Diode/RConn1 -- +/RConn1
  IGBT1/LConn1 -- Diode1/RConn1 -- -/RConn1
  IGBT2/RConn1 -- IGBT1/RConn1 -- Diode/LConn1 -- Diode1/LConn1

== system threephase_matrix_converter/Matrix Converter IGBTs/S2 ==
  g : Inport
  Diode : powerlib/Power Electronics/Diode  Ron=0.001  Lon=0  Vf=0  IC=0  UseSnubber=off  Rs=1e4  Cs=250e-9  Measurements=off
  Diode1 : powerlib/Power Electronics/Diode  Ron=0.001  Lon=0  Vf=0  IC=0  UseSnubber=off  Rs=1e4  Cs=250e-9  Measurements=off
  IGBT1 : powerlib/Power Electronics/IGBT  Ron=0.001  Lon=0  Vf=1  Tf=1e-6  Tt=2e-6  IC=0  Rs=1e5  Cs=inf  Measurements=off
  IGBT2 : powerlib/Power Electronics/IGBT  Ron=0.001  Lon=0  Vf=1  Tf=1e-6  Tt=2e-6  IC=0  Rs=1e5  Cs=inf  Measurements=off
  + : PMIOPort  Port=1  Side=Left
  - : PMIOPort  Port=2  Side=Right
  wires:
  g/1 -> IGBT1/1, IGBT2/1
  connections:
  Diode1/LConn1 -- IGBT1/RConn1 -- IGBT2/RConn1 -- Diode/LConn1
  Diode1/RConn1 -- IGBT1/LConn1 -- -/RConn1
  Diode/RConn1 -- IGBT2/LConn1 -- +/RConn1

== system threephase_matrix_converter/Matrix Converter IGBTs/S3 ==
  g : Inport
  Diode : powerlib/Power Electronics/Diode  Ron=0.001  Lon=0  Vf=0  IC=0  UseSnubber=off  Rs=1e4  Cs=250e-9  Measurements=off
  Diode1 : powerlib/Power Electronics/Diode  Ron=0.001  Lon=0  Vf=0  IC=0  UseSnubber=off  Rs=1e4  Cs=250e-9  Measurements=off
  IGBT1 : powerlib/Power Electronics/IGBT  Ron=0.001  Lon=0  Vf=1  Tf=1e-6  Tt=2e-6  IC=0  Rs=1e5  Cs=inf  Measurements=off
  IGBT2 : powerlib/Power Electronics/IGBT  Ron=0.001  Lon=0  Vf=1  Tf=1e-6  Tt=2e-6  IC=0  Rs=1e5  Cs=inf  Measurements=off
  + : PMIOPort  Port=1  Side=Left
  - : PMIOPort  Port=2  Side=Right
  wires:
  g/1 -> IGBT2/1, IGBT1/1
  connections:
  +/RConn1 -- IGBT2/LConn1 -- Diode/RConn1
  -/RConn1 -- IGBT1/LConn1 -- Diode1/RConn1
  Diode/LConn1 -- IGBT2/RConn1 -- IGBT1/RConn1 -- Diode1/LConn1

== system threephase_matrix_converter/Matrix Converter IGBTs/S4 ==
  g : Inport
  Diode : powerlib/Power Electronics/Diode  Ron=0.001  Lon=0  Vf=0  IC=0  UseSnubber=off  Rs=1e4  Cs=250e-9  Measurements=off
  Diode1 : powerlib/Power Electronics/Diode  Ron=0.001  Lon=0  Vf=0  IC=0  UseSnubber=off  Rs=1e4  Cs=250e-9  Measurements=off
  IGBT1 : powerlib/Power Electronics/IGBT  Ron=0.001  Lon=0  Vf=1  Tf=1e-6  Tt=2e-6  IC=0  Rs=1e5  Cs=inf  Measurements=off
  IGBT2 : powerlib/Power Electronics/IGBT  Ron=0.001  Lon=0  Vf=1  Tf=1e-6  Tt=2e-6  IC=0  Rs=1e5  Cs=inf  Measurements=off
  + : PMIOPort  Port=1  Side=Left
  - : PMIOPort  Port=2  Side=Right
  wires:
  g/1 -> IGBT1/1, IGBT2/1
  connections:
  Diode1/LConn1 -- IGBT1/RConn1 -- IGBT2/RConn1 -- Diode/LConn1
  Diode1/RConn1 -- IGBT1/LConn1 -- -/RConn1
  Diode/RConn1 -- IGBT2/LConn1 -- +/RConn1

== system threephase_matrix_converter/Matrix Converter IGBTs/S5 ==
  g : Inport
  Diode : powerlib/Power Electronics/Diode  Ron=0.001  Lon=0  Vf=0  IC=0  UseSnubber=off  Rs=1e4  Cs=250e-9  Measurements=off
  Diode1 : powerlib/Power Electronics/Diode  Ron=0.001  Lon=0  Vf=0  IC=0  UseSnubber=off  Rs=1e4  Cs=250e-9  Measurements=off
  IGBT1 : powerlib/Power Electronics/IGBT  Ron=0.001  Lon=0  Vf=1  Tf=1e-6  Tt=2e-6  IC=0  Rs=1e5  Cs=inf  Measurements=off
  IGBT2 : powerlib/Power Electronics/IGBT  Ron=0.001  Lon=0  Vf=1  Tf=1e-6  Tt=2e-6  IC=0  Rs=1e5  Cs=inf  Measurements=off
  + : PMIOPort  Port=1  Side=Left
  - : PMIOPort  Port=2  Side=Right
  wires:
  g/1 -> IGBT2/1, IGBT1/1
  connections:
  +/RConn1 -- IGBT2/LConn1 -- Diode/RConn1
  -/RConn1 -- IGBT1/LConn1 -- Diode1/RConn1
  Diode/LConn1 -- IGBT2/RConn1 -- IGBT1/RConn1 -- Diode1/LConn1

== system threephase_matrix_converter/Matrix Converter IGBTs/S6 ==
  g : Inport
  Diode : powerlib/Power Electronics/Diode  Ron=0.001  Lon=0  Vf=0  IC=0  UseSnubber=off  Rs=1e4  Cs=250e-9  Measurements=off
  Diode1 : powerlib/Power Electronics/Diode  Ron=0.001  Lon=0  Vf=0  IC=0  UseSnubber=off  Rs=1e4  Cs=250e-9  Measurements=off
  IGBT1 : powerlib/Power Electronics/IGBT  Ron=0.001  Lon=0  Vf=1  Tf=1e-6  Tt=2e-6  IC=0  Rs=1e5  Cs=inf  Measurements=off
  IGBT2 : powerlib/Power Electronics/IGBT  Ron=0.001  Lon=0  Vf=1  Tf=1e-6  Tt=2e-6  IC=0  Rs=1e5  Cs=inf  Measurements=off
  + : PMIOPort  Port=1  Side=Left
  - : PMIOPort  Port=2  Side=Right
  wires:
  g/1 -> IGBT1/1, IGBT2/1
  connections:
  Diode1/LConn1 -- IGBT1/RConn1 -- IGBT2/RConn1 -- Diode/LConn1
  Diode1/RConn1 -- IGBT1/LConn1 -- -/RConn1
  Diode/RConn1 -- IGBT2/LConn1 -- +/RConn1

== system threephase_matrix_converter/Matrix Converter IGBTs/S7 ==
  g : Inport
  Diode : powerlib/Power Electronics/Diode  Ron=0.001  Lon=0  Vf=0  IC=0  UseSnubber=off  Rs=1e4  Cs=250e-9  Measurements=off
  Diode1 : powerlib/Power Electronics/Diode  Ron=0.001  Lon=0  Vf=0  IC=0  UseSnubber=off  Rs=1e4  Cs=250e-9  Measurements=off
  IGBT1 : powerlib/Power Electronics/IGBT  Ron=0.001  Lon=0  Vf=1  Tf=1e-6  Tt=2e-6  IC=0  Rs=1e5  Cs=inf  Measurements=off
  IGBT2 : powerlib/Power Electronics/IGBT  Ron=0.001  Lon=0  Vf=1  Tf=1e-6  Tt=2e-6  IC=0  Rs=1e5  Cs=inf  Measurements=off
  + : PMIOPort  Port=1  Side=Left
  - : PMIOPort  Port=2  Side=Right
  wires:
  g/1 -> IGBT2/1, IGBT1/1
  connections:
  +/RConn1 -- IGBT2/LConn1 -- Diode/RConn1
  -/RConn1 -- IGBT1/LConn1 -- Diode1/RConn1
  Diode/LConn1 -- IGBT2/RConn1 -- IGBT1/RConn1 -- Diode1/LConn1

== system threephase_matrix_converter/Matrix Converter IGBTs/S8 ==
  g : Inport
  Diode : powerlib/Power Electronics/Diode  Ron=0.001  Lon=0  Vf=0  IC=0  UseSnubber=off  Rs=1e4  Cs=250e-9  Measurements=off
  Diode1 : powerlib/Power Electronics/Diode  Ron=0.001  Lon=0  Vf=0  IC=0  UseSnubber=off  Rs=1e4  Cs=250e-9  Measurements=off
  IGBT1 : powerlib/Power Electronics/IGBT  Ron=0.001  Lon=0  Vf=1  Tf=1e-6  Tt=2e-6  IC=0  Rs=1e5  Cs=inf  Measurements=off
  IGBT2 : powerlib/Power Electronics/IGBT  Ron=0.001  Lon=0  Vf=1  Tf=1e-6  Tt=2e-6  IC=0  Rs=1e5  Cs=inf  Measurements=off
  + : PMIOPort  Port=1  Side=Left
  - : PMIOPort  Port=2  Side=Right
  wires:
  g/1 -> IGBT1/1, IGBT2/1
  connections:
  Diode1/LConn1 -- IGBT1/RConn1 -- IGBT2/RConn1 -- Diode/LConn1
  Diode1/RConn1 -- IGBT1/LConn1 -- -/RConn1
  Diode/RConn1 -- IGBT2/LConn1 -- +/RConn1

== system threephase_matrix_converter/Matrix Converter IGBTs/S9 ==
  g : Inport
  Diode : powerlib/Power Electronics/Diode  Ron=0.001  Lon=0  Vf=0  IC=0  UseSnubber=off  Rs=1e4  Cs=250e-9  Measurements=off
  Diode1 : powerlib/Power Electronics/Diode  Ron=0.001  Lon=0  Vf=0  IC=0  UseSnubber=off  Rs=1e4  Cs=250e-9  Measurements=off
  IGBT1 : powerlib/Power Electronics/IGBT  Ron=0.001  Lon=0  Vf=1  Tf=1e-6  Tt=2e-6  IC=0  Rs=1e5  Cs=inf  Measurements=off
  IGBT2 : powerlib/Power Electronics/IGBT  Ron=0.001  Lon=0  Vf=1  Tf=1e-6  Tt=2e-6  IC=0  Rs=1e5  Cs=inf  Measurements=off
  + : PMIOPort  Port=1  Side=Left
  - : PMIOPort  Port=2  Side=Right
  wires:
  g/1 -> IGBT2/1, IGBT1/1
  connections:
  +/RConn1 -- IGBT2/LConn1 -- Diode/RConn1
  -/RConn1 -- IGBT1/LConn1 -- Diode1/RConn1
  Diode/LConn1 -- IGBT2/RConn1 -- IGBT1/RConn1 -- Diode1/LConn1

== system threephase_matrix_converter/IGBT Matrix Converter SVM Symmetric Switching/SVM Inversion symmetric sequence/Calculate duty-cycles ==
  deg_mag : Inport
  Trigger : TriggerPort
  Constant : Constant  Value=pi/3
  Constant1 : Constant
  Demux : Demux  Outputs=2
  Mux : Mux  Inputs=2
  Mux1 : Mux  Inputs=2
  Product : Product  Inputs=**  RndMeth=Zero
  Sum : Sum  Inputs=+-
  Sum of Elements : Sum  Inputs=+
  Sum1 : Sum  Inputs=-+
  Sum2 : Sum  Inputs=-+
  Trigonometric Function : Trigonometry  Operator=cos
  Trigonometric Function1 : Trigonometry
  deg2rad : Gain  Gain=pi/180
  deg2rad1 : Gain  Gain=0.5/0.866
  d1_d2_d0 : Outport
  wires:
  Sum of Elements/1 -> Sum2/1
  Constant1/1 -> Sum2/2
  Sum2/1 -> Mux1/2  "d0"
  Mux1/1 -> d1_d2_d0/1
  Product/1 -> Sum of Elements/1, Mux1/1  "d1 d2"
  Constant/1 -> Sum1/2
  Mux/1 -> Trigonometric Function1/1, Trigonometric Function/1
  Sum1/1 -> Mux/2
  deg2rad/1 -> Sum1/1, Mux/1  "theta"
  Sum/1 -> Product/1
  Trigonometric Function1/1 -> deg2rad1/1
  Trigonometric Function/1 -> Sum/1
  Demux/2 -> Product/2  "mag"
  Demux/1 -> deg2rad/1
  deg_mag/1 -> Demux/1
  deg2rad1/1 -> Sum/2

== system threephase_matrix_converter/IGBT Matrix Converter SVM Symmetric Switching/SVM Inversion symmetric sequence/Triggered Subsystem ==
  In1 : Inport
  Trigger : TriggerPort
  Out1 : Outport
  wires:
  In1/1 -> Out1/1

== system threephase_matrix_converter/IGBT Matrix Converter SVM Symmetric Switching/SVM Inversion symmetric sequence/abc 2 alpha-beta ==
  Vabc : Inport
  Demux : Demux  Outputs=3
  Gain : Gain  Gain=1/2  SaturateOnIntegerOverflow=on  OutDataTypeStr=Inherit: Same as input  ParamDataTypeStr=Inherit: Same as input
  Gain1 : Gain  Gain=1/2  SaturateOnIntegerOverflow=on  OutDataTypeStr=Inherit: Same as input  ParamDataTypeStr=Inherit: Same as input
  Gain2 : Gain  Gain=sqrt(2/3)  SaturateOnIntegerOverflow=on  OutDataTypeStr=Inherit: Same as input  ParamDataTypeStr=Inherit: Same as input
  Gain3 : Gain  Gain=sqrt(3)/2  SaturateOnIntegerOverflow=on  OutDataTypeStr=Inherit: Same as input  ParamDataTypeStr=Inherit: Same as input
  Gain4 : Gain  Gain=sqrt(3)/2  SaturateOnIntegerOverflow=on  OutDataTypeStr=Inherit: Same as input  ParamDataTypeStr=Inherit: Same as input
  Gain5 : Gain  Gain=sqrt(2/3)  SaturateOnIntegerOverflow=on  OutDataTypeStr=Inherit: Same as input  ParamDataTypeStr=Inherit: Same as input
  Sum : Sum  Inputs=+--  SaturateOnIntegerOverflow=on  InputSameDT=on  OutDataTypeStr=Inherit: Same as first input
  Sum1 : Sum  Inputs=+-  SaturateOnIntegerOverflow=on  InputSameDT=on  OutDataTypeStr=Inherit: Same as first input
  Valpha : Outport
  Vbeta : Outport  Port=2
  wires:
  Gain5/1 -> Vbeta/1
  Gain2/1 -> Valpha/1
  Vabc/1 -> Demux/1
  Gain3/1 -> Sum1/1
  Gain4/1 -> Sum1/2
  Sum1/1 -> Gain5/1
  Sum/1 -> Gain2/1
  Gain1/1 -> Sum/3
  Gain/1 -> Sum/2
  Demux/1 -> Sum/1
  Demux/2 -> Gain/1, Gain3/1
  Demux/3 -> Gain1/1, Gain4/1

== system threephase_matrix_converter/IGBT Matrix Converter SVM Symmetric Switching/SVM Inversion symmetric sequence/alpha-beta 2 deg-mag ==
  Valpha : Inport
  Vbeta : Inport  Port=2
  Math Function : Math  Operator=square  SaturateOnIntegerOverflow=on
  Math Function1 : Math  Operator=sqrt  SaturateOnIntegerOverflow=on
  Mux1 : Mux  Inputs=2
  Sum of Elements : Sum  Inputs=+
  Trigonometric Function : Trigonometry  Operator=atan2
  rad2deg : Gain  Gain=180/pi  SaturateOnIntegerOverflow=on  OutDataTypeStr=Inherit: Same as input  ParamDataTypeStr=Inherit: Same as input
  Vdeg : Outport
  Vmag : Outport  Port=2
  wires:
  Math Function1/1 -> Vmag/1
  rad2deg/1 -> Vdeg/1
  Vbeta/1 -> Mux1/2, Trigonometric Function/1
  Sum of Elements/1 -> Math Function1/1
  Math Function/1 -> Sum of Elements/1
  Mux1/1 -> Math Function/1
  Valpha/1 -> Mux1/1, Trigonometric Function/2
  Trigonometric Function/1 -> rad2deg/1

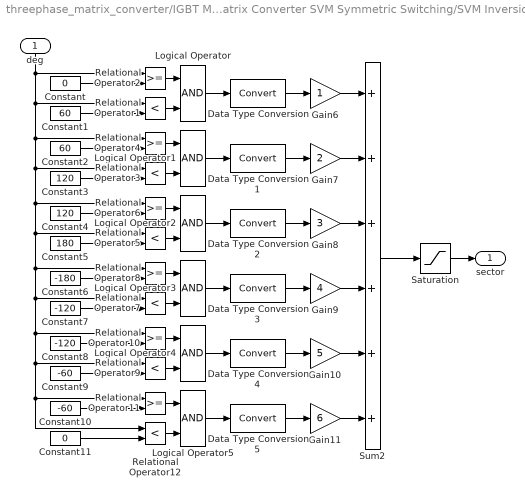
== system threephase_matrix_converter/IGBT Matrix Converter SVM Symmetric Switching/SVM Inversion symmetric sequence/sector ==
  deg : Inport
  Constant : Constant  Value=0
  Constant1 : Constant  Value=60
  Constant10 : Constant  Value=-60
  Constant11 : Constant  Value=0
  Constant2 : Constant  Value=60
  Constant3 : Constant  Value=120
  Constant4 : Constant  Value=120
  Constant5 : Constant  Value=180
  Constant6 : Constant  Value=-180
  Constant7 : Constant  Value=-120
  Constant8 : Constant  Value=-120
  Constant9 : Constant  Value=-60
  Data Type Conversion{,1..5} (6 alike) : DataTypeConversion  SaturateOnIntegerOverflow=on  RndMeth=Zero
  Gain10 : Gain  Gain=5  SaturateOnIntegerOverflow=on  OutDataTypeStr=Inherit: Same as input  ParamDataTypeStr=Inherit: Same as input
  Gain11 : Gain  Gain=6  SaturateOnIntegerOverflow=on  OutDataTypeStr=Inherit: Same as input  ParamDataTypeStr=Inherit: Same as input
  Gain6 : Gain  SaturateOnIntegerOverflow=on  OutDataTypeStr=Inherit: Same as input  ParamDataTypeStr=Inherit: Same as input
  Gain7 : Gain  Gain=2  SaturateOnIntegerOverflow=on  OutDataTypeStr=Inherit: Same as input  ParamDataTypeStr=Inherit: Same as input
  Gain8 : Gain  Gain=3  SaturateOnIntegerOverflow=on  OutDataTypeStr=Inherit: Same as input  ParamDataTypeStr=Inherit: Same as input
  Gain9 : Gain  Gain=4  SaturateOnIntegerOverflow=on  OutDataTypeStr=Inherit: Same as input  ParamDataTypeStr=Inherit: Same as input
  Logical Operator{,1..5} (6 alike) : Logic
  Relational Operator{1,3,5,7,9,12} (6 alike) : RelationalOperator  Operator=<  InputSameDT=on
  Relational Operator{2,4,6,8,10..11} (6 alike) : RelationalOperator  InputSameDT=on
  Saturation : Saturate  UpperLimit=6  LowerLimit=1
  Sum2 : Sum  Inputs=++++++  SaturateOnIntegerOverflow=on  InputSameDT=on  OutDataTypeStr=Inherit: Same as first input
  sector : Outport
  wires:
  Saturation/1 -> sector/1
  deg/1 -> Relational Operator2/1, Relational Operator1/1, Relational Operator4/1, Relational Operator3/1, Relational Operator6/1, Relational Operator5/1, Relational Operator8/1, Relational Operator7/1, Relational Operator10/1, Relational Operator9/1, Relational Operator11/1, Relational Operator12/1
  Data Type Conversion5/1 -> Gain11/1
  Data Type Conversion4/1 -> Gain10/1
  Data Type Conversion3/1 -> Gain9/1
  Data Type Conversion2/1 -> Gain8/1
  Data Type Conversion1/1 -> Gain7/1
  Data Type Conversion/1 -> Gain6/1
  Relational Operator2/1 -> Logical Operator/1
  Relational Operator1/1 -> Logical Operator/2
  Logical Operator/1 -> Data Type Conversion/1
  Constant/1 -> Relational Operator2/2
  Constant1/1 -> Relational Operator1/2
  Relational Operator4/1 -> Logical Operator1/1
  Relational Operator3/1 -> Logical Operator1/2
  Logical Operator1/1 -> Data Type Conversion1/1
  Constant2/1 -> Relational Operator4/2
  Constant3/1 -> Relational Operator3/2
  Relational Operator6/1 -> Logical Operator2/1
  Relational Operator5/1 -> Logical Operator2/2
  Logical Operator2/1 -> Data Type Conversion2/1
  Constant4/1 -> Relational Operator6/2
  Constant5/1 -> Relational Operator5/2
  Relational Operator8/1 -> Logical Operator3/1
  Relational Operator7/1 -> Logical Operator3/2
  Logical Operator3/1 -> Data Type Conversion3/1
  Constant6/1 -> Relational Operator8/2
  Constant7/1 -> Relational Operator7/2
  Relational Operator10/1 -> Logical Operator4/1
  Relational Operator9/1 -> Logical Operator4/2
  Logical Operator4/1 -> Data Type Conversion4/1
  Constant8/1 -> Relational Operator10/2
  Constant9/1 -> Relational Operator9/2
  Relational Operator11/1 -> Logical Operator5/1
  Relational Operator12/1 -> Logical Operator5/2
  Logical Operator5/1 -> Data Type Conversion5/1
  Constant10/1 -> Relational Operator11/2
  Constant11/1 -> Relational Operator12/2
  Gain6/1 -> Sum2/1
  Gain7/1 -> Sum2/2
  Gain8/1 -> Sum2/3
  Gain9/1 -> Sum2/4
  Gain10/1 -> Sum2/5
  Gain11/1 -> Sum2/6
  Sum2/1 -> Saturation/1

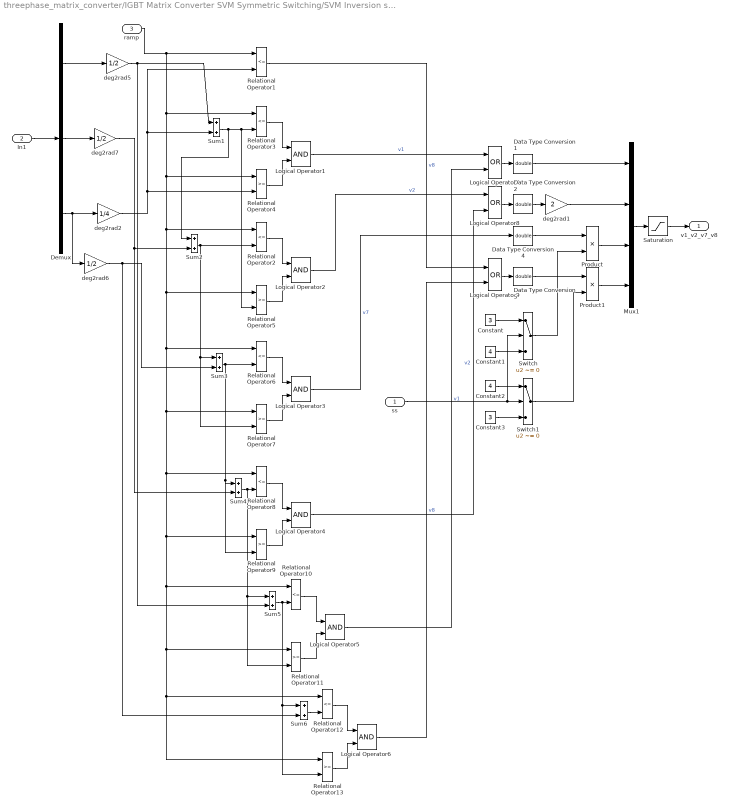
== system threephase_matrix_converter/IGBT Matrix Converter SVM Symmetric Switching/SVM Inversion symmetric sequence/symmetric sequence ==
  ss : Inport
  In1 : Inport  Port=2
  ramp : Inport  Port=3
  Constant : Constant  Value=3
  Constant1 : Constant  Value=4
  Constant2 : Constant  Value=4
  Constant3 : Constant  Value=3
  Data Type Conversion{1..2,4..5} (4 alike) : DataTypeConversion  OutDataTypeStr=double
  Demux : Demux  Outputs=3
  Logical Operator{1..6} (6 alike) : Logic  AllPortsSameDT=off  OutDataTypeStr=boolean
  Logical Operator7 : Logic  Operator=OR  AllPortsSameDT=off  OutDataTypeStr=boolean
  Logical Operator8 : Logic  Operator=OR  AllPortsSameDT=off  OutDataTypeStr=boolean
  Logical Operator9 : Logic  Operator=OR  AllPortsSameDT=off  OutDataTypeStr=boolean
  Mux1 : Mux
  Product : Product  RndMeth=Zero
  Product1 : Product  RndMeth=Zero
  Relational Operator{1..3,6,8,10,12} (7 alike) : RelationalOperator  Operator=<=  InputSameDT=on
  Relational Operator{4..5,7,9,11,13} (6 alike) : RelationalOperator  InputSameDT=on
  Saturation : Saturate  UpperLimit=4  LowerLimit=1
  Sum{1..6} (6 alike) : Sum
  Switch : Switch  Criteria=u2 ~= 0
  Switch1 : Switch  Criteria=u2 ~= 0
  deg2rad1 : Gain  Gain=2
  deg2rad2 : Gain  Gain=1/4
  deg2rad5 : Gain  Gain=1/2
  deg2rad6 : Gain  Gain=1/2
  deg2rad7 : Gain  Gain=1/2
  v1_v2_v7_v8 : Outport
  wires:
  ss/1 -> Switch/2, Switch1/2
  Switch1/1 -> Product1/2
  Switch/1 -> Product/2
  Constant2/1 -> Switch1/1
  Constant3/1 -> Switch1/3
  Constant/1 -> Switch/1
  Constant1/1 -> Switch/3
  Product1/1 -> Mux1/4
  Product/1 -> Mux1/3
  Data Type Conversion5/1 -> Product1/1
  Data Type Conversion4/1 -> Product/1
  Data Type Conversion2/1 -> deg2rad1/1
  Data Type Conversion1/1 -> Mux1/1
  Logical Operator7/1 -> Data Type Conversion1/1
  Relational Operator1/1 -> Logical Operator9/1  "v8"
  Logical Operator1/1 -> Logical Operator7/1  "v1"
  Logical Operator6/1 -> Logical Operator9/2  "v8"
  Sum6/1 -> Relational Operator12/2
  Relational Operator13/1 -> Logical Operator6/2
  Relational Operator12/1 -> Logical Operator6/1
  Logical Operator5/1 -> Logical Operator7/2  "v1"
  Sum5/1 -> Relational Operator13/2, Sum6/1, Relational Operator10/2
  Relational Operator11/1 -> Logical Operator5/2
  Relational Operator10/1 -> Logical Operator5/1
  Logical Operator4/1 -> Logical Operator8/2  "v2"
  deg2rad7/1 -> Sum2/2, Sum4/2
  Demux/2 -> deg2rad7/1
  Sum4/1 -> Sum5/1, Relational Operator11/2, Relational Operator8/2
  Relational Operator9/1 -> Logical Operator4/2
  Relational Operator8/1 -> Logical Operator4/1
  deg2rad6/1 -> Sum6/2, Sum3/2
  Sum3/1 -> Relational Operator9/2, Sum4/1, Relational Operator6/2
  Logical Operator3/1 -> Data Type Conversion4/1  "v7"
  Relational Operator7/1 -> Logical Operator3/2
  Relational Operator6/1 -> Logical Operator3/1
  Logical Operator2/1 -> Logical Operator8/1  "v2"
  Sum2/1 -> Relational Operator7/2, Sum3/1, Relational Operator2/2
  Relational Operator5/1 -> Logical Operator2/2
  Relational Operator2/1 -> Logical Operator2/1
  deg2rad5/1 -> Sum5/2, Sum1/1
  Demux/1 -> deg2rad5/1
  deg2rad2/1 -> Sum1/2, Relational Operator1/2, Relational Operator4/2
  Sum1/1 -> Sum2/1, Relational Operator5/2, Relational Operator3/2
  Relational Operator4/1 -> Logical Operator1/2
  Relational Operator3/1 -> Logical Operator1/1
  Saturation/1 -> v1_v2_v7_v8/1
  Logical Operator9/1 -> Data Type Conversion5/1
  Logical Operator8/1 -> Data Type Conversion2/1
  deg2rad1/1 -> Mux1/2
  In1/1 -> Demux/1
  ramp/1 -> Relational Operator1/1, Relational Operator13/1, Relational Operator12/1, Relational Operator11/1, Relational Operator10/1, Relational Operator9/1, Relational Operator8/1, Relational Operator7/1, Relational Operator6/1, Relational Operator5/1, Relational Operator2/1, Relational Operator4/1, Relational Operator3/1
  Mux1/1 -> Saturation/1
  Demux/3 -> deg2rad6/1, deg2rad2/1

== system threephase_matrix_converter/IGBT Matrix Converter SVM Symmetric Switching/SVM Rectification symmetric sequence/Calculate duty-cycles ==
  deg_mag : Inport
  Trigger : TriggerPort
  Constant : Constant  Value=pi/3
  Constant1 : Constant
  Demux : Demux  Outputs=2
  Mux : Mux  Inputs=2
  Mux1 : Mux  Inputs=2
  Product : Product  Inputs=**  RndMeth=Zero
  Sum : Sum  Inputs=+-
  Sum of Elements : Sum  Inputs=+
  Sum1 : Sum  Inputs=-+
  Sum2 : Sum  Inputs=-+
  Trigonometric Function : Trigonometry  Operator=cos
  Trigonometric Function1 : Trigonometry
  deg2rad : Gain  Gain=pi/180
  deg2rad1 : Gain  Gain=0.5/0.866
  d1_d2_d0 : Outport
  wires:
  Sum of Elements/1 -> Sum2/1
  Constant1/1 -> Sum2/2
  Sum2/1 -> Mux1/2  "d0"
  Mux1/1 -> d1_d2_d0/1
  Product/1 -> Sum of Elements/1, Mux1/1  "d1 d2"
  Constant/1 -> Sum1/2
  Mux/1 -> Trigonometric Function1/1, Trigonometric Function/1
  Sum1/1 -> Mux/2
  deg2rad/1 -> Sum1/1, Mux/1  "theta"
  Sum/1 -> Product/1
  deg2rad1/1 -> Sum/2
  Trigonometric Function1/1 -> deg2rad1/1
  Trigonometric Function/1 -> Sum/1
  Demux/2 -> Product/2  "mag"
  Demux/1 -> deg2rad/1
  deg_mag/1 -> Demux/1

== system threephase_matrix_converter/IGBT Matrix Converter SVM Symmetric Switching/SVM Rectification symmetric sequence/Triggered Subsystem ==
  In1 : Inport
  Trigger : TriggerPort
  Out1 : Outport
  wires:
  In1/1 -> Out1/1

== system threephase_matrix_converter/IGBT Matrix Converter SVM Symmetric Switching/SVM Rectification symmetric sequence/abc 2 alpha-beta ==
  Vabc : Inport
  Demux : Demux  Outputs=3
  Gain : Gain  Gain=1/2  SaturateOnIntegerOverflow=on  OutDataTypeStr=Inherit: Same as input  ParamDataTypeStr=Inherit: Same as input
  Gain1 : Gain  Gain=1/2  SaturateOnIntegerOverflow=on  OutDataTypeStr=Inherit: Same as input  ParamDataTypeStr=Inherit: Same as input
  Gain2 : Gain  Gain=sqrt(2/3)  SaturateOnIntegerOverflow=on  OutDataTypeStr=Inherit: Same as input  ParamDataTypeStr=Inherit: Same as input
  Gain3 : Gain  Gain=sqrt(3)/2  SaturateOnIntegerOverflow=on  OutDataTypeStr=Inherit: Same as input  ParamDataTypeStr=Inherit: Same as input
  Gain4 : Gain  Gain=sqrt(3)/2  SaturateOnIntegerOverflow=on  OutDataTypeStr=Inherit: Same as input  ParamDataTypeStr=Inherit: Same as input
  Gain5 : Gain  Gain=sqrt(2/3)  SaturateOnIntegerOverflow=on  OutDataTypeStr=Inherit: Same as input  ParamDataTypeStr=Inherit: Same as input
  Sum : Sum  Inputs=+--  SaturateOnIntegerOverflow=on  InputSameDT=on  OutDataTypeStr=Inherit: Same as first input
  Sum1 : Sum  Inputs=+-  SaturateOnIntegerOverflow=on  InputSameDT=on  OutDataTypeStr=Inherit: Same as first input
  Valpha : Outport
  Vbeta : Outport  Port=2
  wires:
  Gain5/1 -> Vbeta/1
  Gain2/1 -> Valpha/1
  Vabc/1 -> Demux/1
  Gain3/1 -> Sum1/1
  Gain4/1 -> Sum1/2
  Sum1/1 -> Gain5/1
  Sum/1 -> Gain2/1
  Gain1/1 -> Sum/3
  Gain/1 -> Sum/2
  Demux/1 -> Sum/1
  Demux/2 -> Gain/1, Gain3/1
  Demux/3 -> Gain1/1, Gain4/1

== system threephase_matrix_converter/IGBT Matrix Converter SVM Symmetric Switching/SVM Rectification symmetric sequence/alpha-beta 2 deg-mag ==
  Valpha : Inport
  Vbeta : Inport  Port=2
  Constant1 : Constant  Value=180
  Constant2 : Constant  Value=-360
  Constant20 : Constant  Value=30
  Math Function : Math  Operator=square  SaturateOnIntegerOverflow=on
  Math Function1 : Math  Operator=sqrt  SaturateOnIntegerOverflow=on
  Mux1 : Mux  Inputs=2
  Relational Operator2 : RelationalOperator  Operator=>  InputSameDT=on
  Sum of Elements : Sum  Inputs=+
  Sum1 : Sum  Inputs=|++
  Sum2 : Sum  Inputs=|++
  Switch : Switch  Criteria=u2 ~= 0
  Trigonometric Function : Trigonometry  Operator=atan2
  rad2deg : Gain  Gain=180/pi  SaturateOnIntegerOverflow=on  OutDataTypeStr=Inherit: Same as input  ParamDataTypeStr=Inherit: Same as input
  Vdeg : Outport
  Vmag : Outport  Port=2
  wires:
  Trigonometric Function/1 -> rad2deg/1
  Valpha/1 -> Trigonometric Function/2, Mux1/1
  Mux1/1 -> Math Function/1
  Math Function/1 -> Sum of Elements/1
  Sum of Elements/1 -> Math Function1/1
  Vbeta/1 -> Trigonometric Function/1, Mux1/2
  Math Function1/1 -> Vmag/1
  rad2deg/1 -> Sum1/1
  Constant20/1 -> Sum1/2
  Sum1/1 -> Relational Operator2/1, Switch/3, Sum2/1
  Relational Operator2/1 -> Switch/2
  Switch/1 -> Vdeg/1
  Constant1/1 -> Relational Operator2/2
  Sum2/1 -> Switch/1
  Constant2/1 -> Sum2/2
